simulink model "Fig338"  (R2014b)
settings: Solver=ode3  StartTime=0.0  StopTime=3  FixedStep=2e-6  RelTol=1e-5
libraries: commfilt2 x2, commutil2 x1, commchan3 x1, commrandsrc2 x1
settings Model: Creator=Dennis Silage  LastModifiedBy=Silage
settings DataIOCC: SignalLoggingSaveFormat=ModelDataLogs
settings OptimizationCC: ExpressionDepthLimit=2147483647  InitFltsAndDblsToZero=on
settings DebuggingCC: UnderspecifiedInitializationDetection=Classic  MergeDetectMultiDrivingBlocksExec=none  SolverPrmCheckMsg=none  FcnCallInpInsideContextMsg=UseLocalSettings  StateNameClashWarn=warning
settings GRTTargetCC: CombineOutputUpdateFcns=off  GRTInterface=on

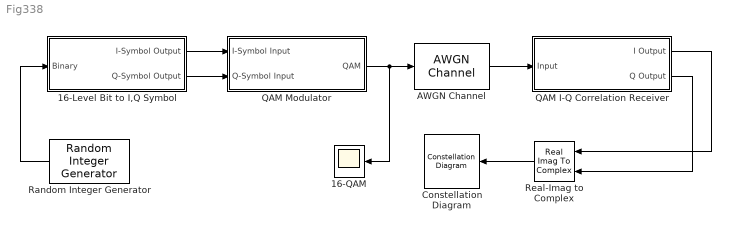
== system Fig338 ==
  16-Level Bit to I,Q Symbol : Subsystem
  16-QAM : Scope
      settings: TimeRange=0.005  YMin=-10  YMax=10  MaxDataPoints=8001
  AWGN Channel : commchan3/AWGN Channel  InputProcessing=Inherited (this choice will be removed - see release notes)  seed=randseed  noiseMode="Signal to noise ratio  (Eb/No)"  EbNodB=50  EsNodB=20  SNRdB=10  bitsPerSym=4  Ps=1.25  Tsym=4e-3  variance=0
  Constellation Diagram : ConstellationDiagram
  QAM I-Q Correlation Receiver : Subsystem
  QAM Modulator : Subsystem
  Random Integer Generator : commrandsrc2/Random Integer Generator  mul=2  seed=randseed  Ts=1e-3  frameBased=off  sampPerFrame=1  orient=off  outDataType=double
  Real-Imag to Complex : RealImagToComplex
  wires:
  QAM Modulator/1(QAM) -> AWGN Channel/1, 16-QAM/1
  Random Integer Generator/1 -> 16-Level Bit to I,Q Symbol/1(Binary)
  AWGN Channel/1 -> QAM I-Q Correlation Receiver/1(Input)
  16-Level Bit to I,Q Symbol/1(I-Symbol Output) -> QAM Modulator/1(I-Symbol Input)
  16-Level Bit to I,Q Symbol/2(Q-Symbol Output) -> QAM Modulator/2(Q-Symbol Input)
  Real-Imag to Complex/1 -> Constellation Diagram/1
  QAM I-Q Correlation Receiver/1(I Output) -> Real-Imag to Complex/1
  QAM I-Q Correlation Receiver/2(Q Output) -> Real-Imag to Complex/2

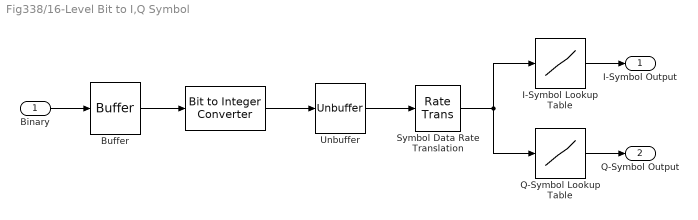
== system Fig338/16-Level Bit to I,Q Symbol ==
  Binary : Inport
  " " : commutil2/Bit to Integer Converter  nbits=4  bitOrder=MSB first  signedOutputValues=Unsigned  outDtype=Inherit via internal rule  outDtypeSigned=Inherit via internal rule
  Buffer : Buffer  N=4  TreatMby1Signals=One channel
  I-Symbol Lookup Table : Lookup_n-D  NumberOfTableDimensions=1  BreakpointsForDimension1=[0,1,2,3,4,5,6,7,8,9,10,11,12,13,14,15]  Table=[-1,-3,-1,-3,1,1,3,3,-1,-1,-3,-3,1,3,1,3]  InternalRulePriority=Speed  RndMeth=Simplest  InputSameDT=on
  Q-Symbol Lookup Table : Lookup_n-D  NumberOfTableDimensions=1  BreakpointsForDimension1=[0,1,2,3,4,5,6,7,8,9,10,11,12,13,14,15]  Table=[1,1,3,3,1,3,1,3,-1,-3,-1,-3,-1,-1,-3,-3]  InternalRulePriority=Speed  RndMeth=Simplest  InputSameDT=on
  Symbol Data Rate Translation : RateTransition  OutPortSampleTime=4e-3
  Unbuffer : Unbuffer  SampleBasedProcessing=Same as frame based
  I-Symbol Output : Outport
  Q-Symbol Output : Outport  Port=2
  wires:
  Symbol Data Rate Translation/1 -> Q-Symbol Lookup Table/1, I-Symbol Lookup Table/1
  Binary/1 -> Buffer/1
  Buffer/1 -> " "/1
  " "/1 -> Unbuffer/1
  Unbuffer/1 -> Symbol Data Rate Translation/1
  I-Symbol Lookup Table/1 -> I-Symbol Output/1
  Q-Symbol Lookup Table/1 -> Q-Symbol Output/1

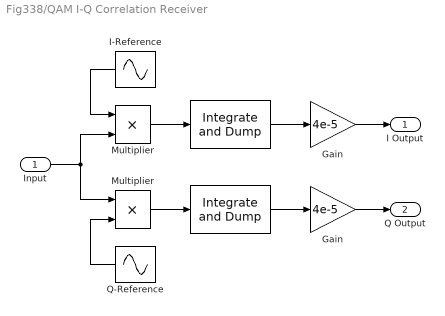
== system Fig338/QAM I-Q Correlation Receiver ==
  Input : Inport
  " " : commfilt2/Integrate and Dump  obssamples=2000  offsetsamples=0  nodump=off  roundingMode=Floor  overflowMode=off
  "  " : commfilt2/Integrate and Dump  obssamples=2000  offsetsamples=0  nodump=off  roundingMode=Floor  overflowMode=off
  Gain : Gain  Gain=4e-5
  "Gain " : Gain  Gain=4e-5
  I-Reference : Sin  Amplitude=5  Frequency=40000*pi  Phase=pi/2  SampleTime=2e-6
  Multiplier : Product  RndMeth=Zero
  "Multiplier " : Product  RndMeth=Zero
  Q-Reference : Sin  Amplitude=5  Frequency=40000*pi  SampleTime=2e-6
  I Output : Outport
  Q Output : Outport  Port=2
  wires:
  "Multiplier "/1 -> " "/1
  Multiplier/1 -> "  "/1
  " "/1 -> Gain/1
  "  "/1 -> "Gain "/1
  I-Reference/1 -> "Multiplier "/1
  Q-Reference/1 -> Multiplier/2
  Input/1 -> "Multiplier "/2, Multiplier/1
  Gain/1 -> I Output/1
  "Gain "/1 -> Q Output/1

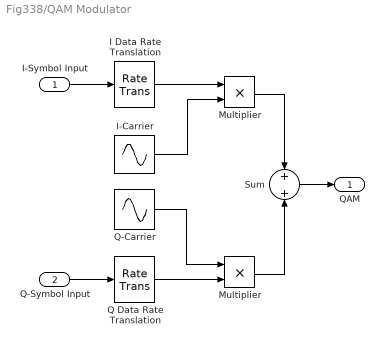
== system Fig338/QAM Modulator ==
  I-Symbol Input : Inport
  Q-Symbol Input : Inport  Port=2
  " Multiplier " : Product  RndMeth=Zero
  I Data Rate Translation : RateTransition  OutPortSampleTime=2e-6
  I-Carrier : Sin  Amplitude=5  Frequency=40000*pi  Phase=pi/2  SampleTime=2e-6  VectorParams1D=off
  Multiplier : Product  RndMeth=Zero
  Q Data Rate Translation : RateTransition  OutPortSampleTime=2e-6
  Q-Carrier : Sin  Amplitude=5  Frequency=40000*pi  SampleTime=2e-6  VectorParams1D=off
  Sum : Sum
  QAM : Outport
  wires:
  I Data Rate Translation/1 -> Multiplier/1
  Q Data Rate Translation/1 -> " Multiplier "/2
  I-Carrier/1 -> Multiplier/2
  Q-Carrier/1 -> " Multiplier "/1
  Multiplier/1 -> Sum/1
  " Multiplier "/1 -> Sum/2
  Sum/1 -> QAM/1
  I-Symbol Input/1 -> I Data Rate Translation/1
  Q-Symbol Input/1 -> Q Data Rate Translation/1
